simulink model "linearizedTurbine_2022b_mdl"  (R2022b)
settings: Solver=ode4  StartTime=0.0  StopTime=150  FixedStep=.001  RelTol=1e-3
undefined symbols (not defined in the file): A, A_F, A_G, B, B_F, B_G, C, C_F, C_G, D, D_F, D_G, F, G, P0
settings Model: Creator=mo780715  LastModifiedBy=mo780715

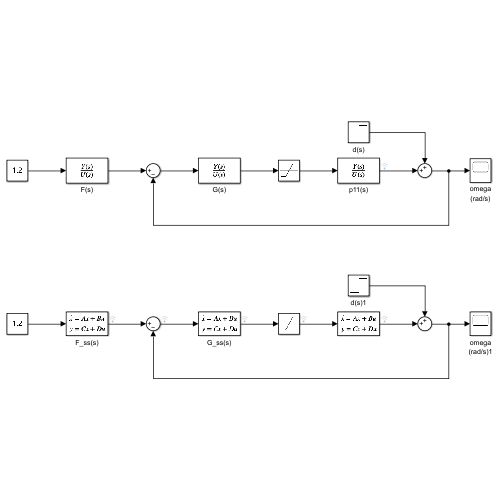
[thumbnail: Simulink's stored preview of the top-level diagram]
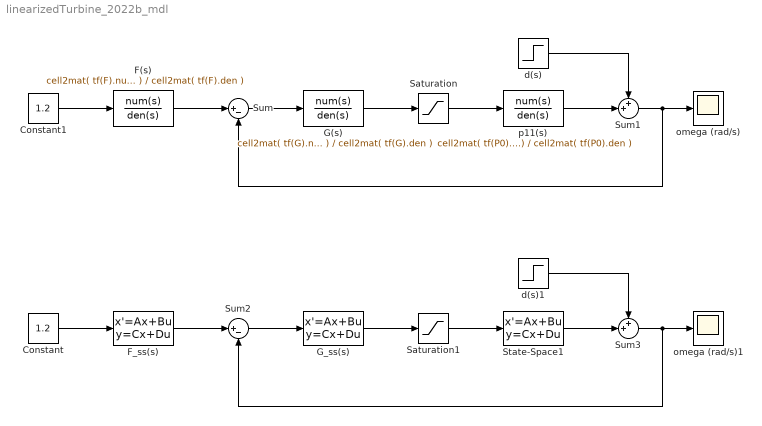
== system linearizedTurbine_2022b_mdl ==
  Constant : Constant  Value=1.2
  Constant1 : Constant  Value=1.2
  F(s) : TransferFcn  Numerator=cell2mat( tf(F).num )  Denominator=cell2mat( tf(F).den )
  F_ss(s) : StateSpace  A=A_F  B=B_F  C=C_F  D=D_F  InitialCondition=0.5/0.4725  ParameterTunability=Optimized
  G(s) : TransferFcn  Numerator=cell2mat( tf(G).num )  Denominator=cell2mat( tf(G).den )
  G_ss(s) : StateSpace  A=A_G  B=B_G  C=C_G  D=D_G  InitialCondition=0  ParameterTunability=Unconstrained
  Saturation : Saturate  UpperLimit=25 * pi/180  LowerLimit=0
  Saturation1 : Saturate  UpperLimit=25 * pi/180  LowerLimit=0
  State-Space1 : StateSpace  A=A  B=B  C=C  D=D  InitialCondition=[0 0.5 0 0 0 0 0 0]  ParameterTunability=Unconstrained
  Sum : Sum  Inputs=|+-
  Sum1 : Sum  Inputs=++|
  Sum2 : Sum  Inputs=|+-
  Sum3 : Sum  Inputs=++|
  d(s) : Step  Time=80  After=0.1  SampleTime=0
  d(s)1 : Step  Time=80  After=0.1  SampleTime=0
  omega (rad/s) : Scope
  omega (rad/s)1 : Scope
  p11(s) : TransferFcn  Numerator=cell2mat( tf(P0).num )  Denominator=cell2mat( tf(P0).den )
  wires:
  Sum1/1 -> omega (rad/s)/1, Sum/2
  F(s)/1 -> Sum/1
  Sum/1 -> G(s)/1
  Constant1/1 -> F(s)/1
  p11(s)/1 -> Sum1/2
  d(s)/1 -> Sum1/1
  G(s)/1 -> Saturation/1
  Saturation/1 -> p11(s)/1
  Constant/1 -> F_ss(s)/1
  d(s)1/1 -> Sum3/1
  Sum3/1 -> omega (rad/s)1/1, Sum2/2
  Sum2/1 -> G_ss(s)/1
  F_ss(s)/1 -> Sum2/1
  State-Space1/1 -> Sum3/2
  Saturation1/1 -> State-Space1/1
  G_ss(s)/1 -> Saturation1/1
